simulink model "cinematico_com_espaco_de_estados"  (R2016a)
settings: Solver=ode45  StartTime=0.0  StopTime=25  FixedStep=0.001  RelTol=1e-3
InitFcn:
  | clear all;
  | Kpx = 10;
  | Kix = 25;
  | Kpy = 10;
  | Kiy = 25;
  | Kvphi = 3;
  | Kpphi = 2.25;
  | 
  | Kem = 0.0059;
  | Kti = 0.0059;
  | Vd = 5.4;
  | R = 1.71;
  | r = 0.072;
  | eta = 0.83;
  | N = 19;
  | 
  | Jw = 8.1e-4
libraries: simulink x1
settings Model: Creator=Pichau  LastModifiedBy=Pichau

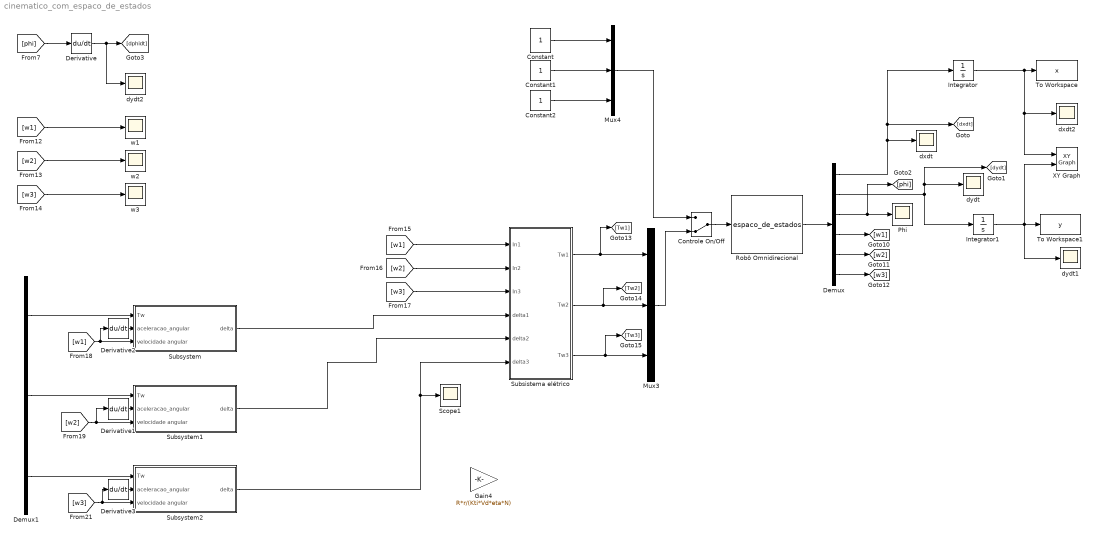
== system cinematico_com_espaco_de_estados ==
  Constant : Constant
  Constant1 : Constant
  Constant2 : Constant
  Controle On/Off : ManualSwitch  CurrentSetting=0
  Demux : Demux  Outputs=6
  Demux1 : Demux  Outputs=3
  Derivative{,1..3} (4 alike) : Derivative
  Gain4 : Gain  Gain=R*r/(Kti*Vd*eta*N)
  Integrator : Integrator  InitialCondition=0.3
  Integrator1 : Integrator
  Mux3 : Mux  Inputs=3
  Mux4 : Mux  Inputs=3
  Phi : Scope
  Robô Omnidirecional : S-Function  FunctionName=espaco_de_estados  Parameters=r,m,Jw,J,L  SFunctionDeploymentMode=off  EnableBusSupport=off  mask{r=0.072, m=1.71, Jw=8.1e-4, J=2.125, L=0.09}
      mask prompts: r "r (m)"; m "m (Kg)"; Jw "Jw (Kg*m^2)"; J "J (Kg*m^2)"; L "L (m)"
      mask Display: image(imread('Robot_omnidirectional_drive.png'));
  Scope1 : Scope
  Subsistema elétrico : Subsystem
  Subsystem : Subsystem
  Subsystem1 : Subsystem
  Subsystem2 : Subsystem
  To Workspace : ToWorkspace  VariableName=x  SaveFormat=Timeseries  SampleTime=-1
  To Workspace1 : ToWorkspace  VariableName=y  SaveFormat=Timeseries  SampleTime=-1
  XY Graph : simulink/Sinks/XY Graph  xmin=-1  xmax=1  ymin=-1  ymax=1  st=-1
  dxdt : Scope
  dxdt2 : Scope
  dydt : Scope
  dydt1 : Scope
  dydt2 : Scope
  w1 : Scope
  w2 : Scope
  w3 : Scope
  wires:
  Robô Omnidirecional/1 -> Demux/1
  Integrator1/1 -> XY Graph/2, To Workspace1/1, dydt1/1
  Integrator/1 -> XY Graph/1, dxdt2/1, To Workspace/1
  Derivative/1 -> dydt2/1, [dphidt]
  Mux3/1 -> Controle On/Off/2
  Controle On/Off/1 -> Robô Omnidirecional/1
  [w3] -> w3/1
  [w2] -> w2/1
  [w1] -> w1/1
  Demux/1 -> [dxdt], Integrator/1, dxdt/1
  Demux/2 -> Integrator1/1, [dydt], dydt/1
  Demux/3 -> Phi/1, [phi]
  [phi] -> Derivative/1
  Demux/4 -> [w1]
  Demux/5 -> [w2]
  Demux/6 -> [w3]
  [w1] -> Subsistema elétrico/1(In1)
  [w2] -> Subsistema elétrico/2(In2)
  [w3] -> Subsistema elétrico/3(In3)
  Subsistema elétrico/3(Tw3) -> [Tw3], Mux3/3
  Subsistema elétrico/2(Tw2) -> [Tw2], Mux3/2
  Subsistema elétrico/1(Tw1) -> [Tw1], Mux3/1
  Mux4/1 -> Controle On/Off/1
  Demux1/1 -> Subsystem/1(Tw)
  Demux1/2 -> Subsystem1/1(Tw)
  Demux1/3 -> Subsystem2/1(Tw)
  Subsystem1/1(delta) -> Subsistema elétrico/5(delta2)
  Subsystem2/1(delta) -> Subsistema elétrico/6(delta3), Scope1/1
  Subsystem/1(delta) -> Subsistema elétrico/4(delta1)
  [w1] -> Derivative2/1, Subsystem/3(velocidade angular)
  [w2] -> Derivative1/1, Subsystem1/3(velocidade angular)
  [w3] -> Derivative3/1, Subsystem2/3(velocidade angular)
  Derivative1/1 -> Subsystem1/2(aceleracao_angular)
  Derivative2/1 -> Subsystem/2(aceleracao_angular)
  Derivative3/1 -> Subsystem2/2(aceleracao_angular)
  Constant/1 -> Mux4/1
  Constant1/1 -> Mux4/2
  Constant2/1 -> Mux4/3

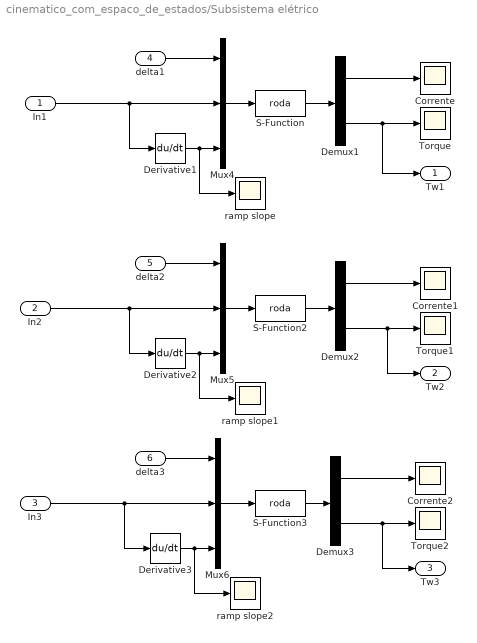
== system cinematico_com_espaco_de_estados/Subsistema elétrico ==
  In1 : Inport
  In2 : Inport  Port=2
  In3 : Inport  Port=3
  delta1 : Inport  Port=4
  delta2 : Inport  Port=5
  delta3 : Inport  Port=6
  Corrente : Scope
  Corrente1 : Scope
  Corrente2 : Scope
  Demux1 : Demux  Outputs=2
  Demux2 : Demux  Outputs=2
  Demux3 : Demux  Outputs=2
  Derivative1 : Derivative
  Derivative2 : Derivative
  Derivative3 : Derivative
  Mux4 : Mux  Inputs=3
  Mux5 : Mux  Inputs=3
  Mux6 : Mux  Inputs=3
  S-Function : S-Function  FunctionName=roda  Parameters=Vd,Vsat,deltaVd,L,Kem,R,Kti,Jm,eta,N  SFunctionDeploymentMode=off  EnableBusSupport=off  mask{Vd=6, Vsat=0.3, deltaVd=0, L=0.00011, Kem=0.0059, R=1.71, Kti=0.0059, Jm=3.88e-7, eta=0.83, N=19}
  S-Function2 : S-Function  FunctionName=roda  Parameters=Vd,Vsat,deltaVd,L,Kem,R,Kti,Jm,eta,N  SFunctionDeploymentMode=off  EnableBusSupport=off  mask{Vd=6, Vsat=0.3, deltaVd=0, L=0.00011, Kem=0.0059, R=1.71, Kti=0.0059, Jm=3.88e-7, eta=0.83, N=19}
  S-Function3 : S-Function  FunctionName=roda  Parameters=Vd,Vsat,deltaVd,L,Kem,R,Kti,Jm,eta,N  SFunctionDeploymentMode=off  EnableBusSupport=off  mask{Vd=6, Vsat=0.3, deltaVd=0, L=0.00011, Kem=0.0059, R=1.71, Kti=0.0059, Jm=3.88e-7, eta=0.83, N=19}
  Torque : Scope
  Torque1 : Scope
  Torque2 : Scope
  ramp slope : Scope
  ramp slope1 : Scope
  ramp slope2 : Scope
  Tw1 : Outport
  Tw2 : Outport  Port=2
  Tw3 : Outport  Port=3
  wires:
  Demux3/1 -> Corrente2/1
  Mux6/1 -> S-Function3/1
  Derivative3/1 -> ramp slope2/1, Mux6/3
  Demux3/2 -> Tw3/1, Torque2/1
  In3/1 -> Mux6/2, Derivative3/1
  S-Function3/1 -> Demux3/1
  delta2/1 -> Mux5/1
  delta3/1 -> Mux6/1
  Mux5/1 -> S-Function2/1
  In2/1 -> Derivative2/1, Mux5/2
  S-Function2/1 -> Demux2/1
  Demux2/1 -> Corrente1/1
  Demux2/2 -> Tw2/1, Torque1/1
  Derivative2/1 -> Mux5/3, ramp slope1/1
  Derivative1/1 -> ramp slope/1, Mux4/3
  In1/1 -> Mux4/2, Derivative1/1
  Demux1/2 -> Tw1/1, Torque/1
  Mux4/1 -> S-Function/1
  S-Function/1 -> Demux1/1
  delta1/1 -> Mux4/1
  Demux1/1 -> Corrente/1

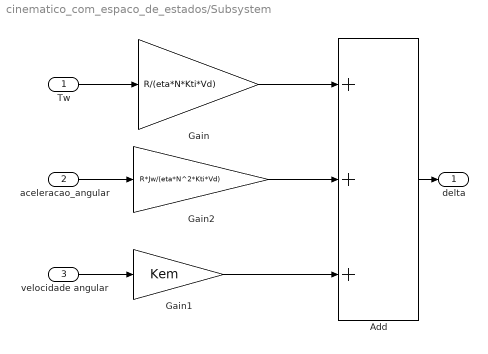
== system cinematico_com_espaco_de_estados/Subsystem ==
  Tw : Inport
  aceleracao_angular : Inport  Port=2
  velocidade angular : Inport  Port=3
  Add : Sum  Inputs=+++
  Gain : Gain  Gain=R/(eta*N*Kti*Vd)
  Gain1 : Gain  Gain=Kem
  Gain2 : Gain  Gain=R*Jw/(eta*N^2*Kti*Vd)
  delta : Outport
  wires:
  aceleracao_angular/1 -> Gain2/1
  velocidade angular/1 -> Gain1/1
  Add/1 -> delta/1
  Tw/1 -> Gain/1
  Gain1/1 -> Add/3
  Gain/1 -> Add/1
  Gain2/1 -> Add/2

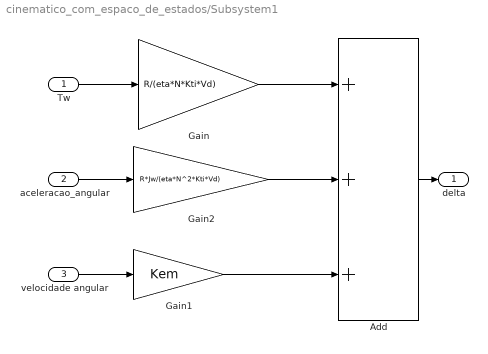
== system cinematico_com_espaco_de_estados/Subsystem1 ==
  Tw : Inport
  aceleracao_angular : Inport  Port=2
  velocidade angular : Inport  Port=3
  Add : Sum  Inputs=+++
  Gain : Gain  Gain=R/(eta*N*Kti*Vd)
  Gain1 : Gain  Gain=Kem
  Gain2 : Gain  Gain=R*Jw/(eta*N^2*Kti*Vd)
  delta : Outport
  wires:
  Gain2/1 -> Add/2
  Gain/1 -> Add/1
  Gain1/1 -> Add/3
  Tw/1 -> Gain/1
  Add/1 -> delta/1
  velocidade angular/1 -> Gain1/1
  aceleracao_angular/1 -> Gain2/1

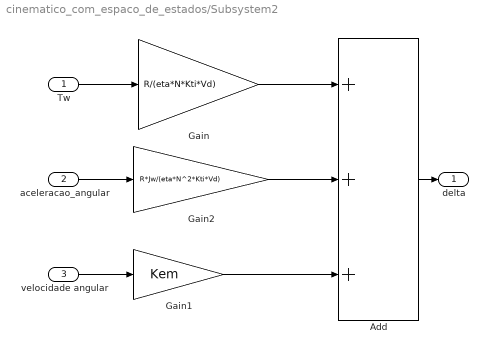
== system cinematico_com_espaco_de_estados/Subsystem2 ==
  Tw : Inport
  aceleracao_angular : Inport  Port=2
  velocidade angular : Inport  Port=3
  Add : Sum  Inputs=+++
  Gain : Gain  Gain=R/(eta*N*Kti*Vd)
  Gain1 : Gain  Gain=Kem
  Gain2 : Gain  Gain=R*Jw/(eta*N^2*Kti*Vd)
  delta : Outport
  wires:
  aceleracao_angular/1 -> Gain2/1
  velocidade angular/1 -> Gain1/1
  Add/1 -> delta/1
  Tw/1 -> Gain/1
  Gain1/1 -> Add/3
  Gain/1 -> Add/1
  Gain2/1 -> Add/2
